simulink model "open_loop"  (R2020b)
settings: Solver=VariableStepAuto  StartTime=0.0  StopTime=50.0  RelTol=1e-3
values from neighbouring files (symbols this model uses):
  K = 1    [lab1.m]    (also in lab1_5.m = i*1.5)
settings Model: Creator=kengoakano  LastModifiedBy=kengoakano

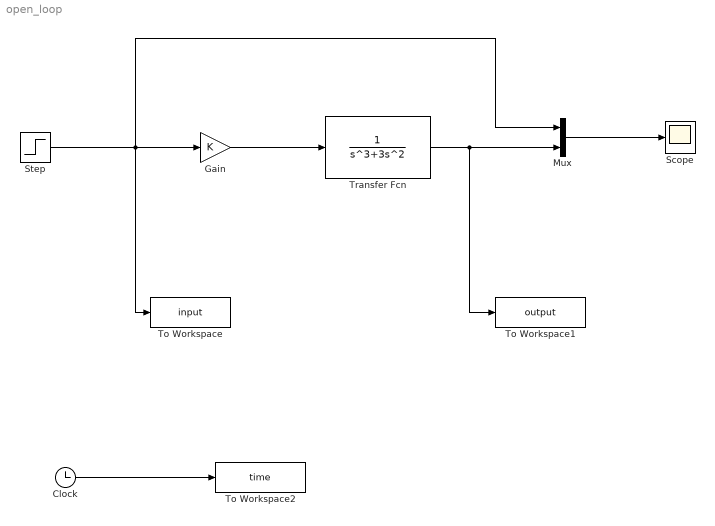
== system open_loop ==
  Clock : Clock
  Gain : Gain  Gain=K
  Mux : Mux  Inputs=2
  Scope : Scope
  Step : Step  SampleTime=0
  To Workspace : ToWorkspace  VariableName=input  SaveFormat=Timeseries  SampleTime=-1
  To Workspace1 : ToWorkspace  VariableName=output  SaveFormat=Timeseries  SampleTime=-1
  To Workspace2 : ToWorkspace  VariableName=time  SaveFormat=Timeseries  SampleTime=-1
  Transfer Fcn : TransferFcn  Denominator=[1 3 0 0]
  wires:
  Gain/1 -> Transfer Fcn/1
  Transfer Fcn/1 -> To Workspace1/1, Mux/2
  Mux/1 -> Scope/1
  Step/1 -> Mux/1, Gain/1, To Workspace/1
  Clock/1 -> To Workspace2/1
